simulink model "aa"  (R2021b)
settings: Solver=FixedStepAuto  StartTime=0.0  StopTime=inf  FixedStep=0.00025  RelTol=1e-3  EnableMultiTasking=on
libraries: arduinolib x11, simulink x7, hdlsllib x6
settings Model: ExtModeTrigDuration=2  Creator=user1  LastModifiedBy=ztaha
settings OptimizationCC: EnhancedBackFolding=on  PassReuseOutputArgsThreshold=0  MaxStackSize=64  OptimizeBlockOrder=speed  DifferentSizesBufferReuse=on  OptimizationCustomize=off
settings DebuggingCC: ParameterTunabilityLossMsg=error  UnconnectedInputMsg=none  UnconnectedOutputMsg=none  UnconnectedLineMsg=none
settings HardwareCC: ProdBitPerInt=16  ProdBitPerPointer=16  ProdBitPerSizeT=16  ProdBitPerPtrDiffT=16  ProdLargestAtomicFloat=None  ProdWordSize=8  ProdHWDeviceType=Atmel->AVR  UseEmbeddedCoderFeatures=off  UseSimulinkCoderFeatures=off
settings SFSimCC: MATLABDynamicMemAlloc=off
settings RTWCC: Description=Embedded Coder  SystemTargetFile=ert.tlc  HardwareBoard=Arduino Mega 2560  TemplateMakefile=ert_default_tmf  Toolchain=Arduino AVR  BuildConfiguration=Faster Runs  DLArmComputeVersion=20.02.1
settings CodeAppCC: ForceParamTrailComments=on  OperatorAnnotations=on  MangleLength=10
settings ERTTargetCC: ERTCustomFileBanners=off  SupportContinuousTime=on  SupportNonInlinedSFcns=on  RemoveResetFunc=off  SupportVariableSizeSignals=on  ModelStepFunctionPrototypeControlCompliant=off  ExtModeTransport=3  ExtModeStaticAlloc=on  ExtModeStaticAllocSize=2048  ExtModeMexFile=ext_xcp  ExtModeIntrfLevel=Level2 - Open

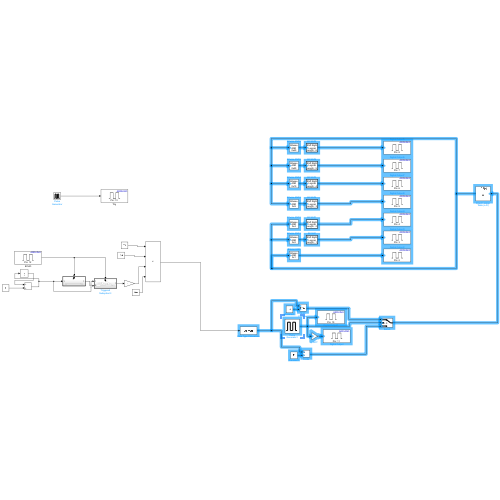
[thumbnail: Simulink's stored preview of the top-level diagram]
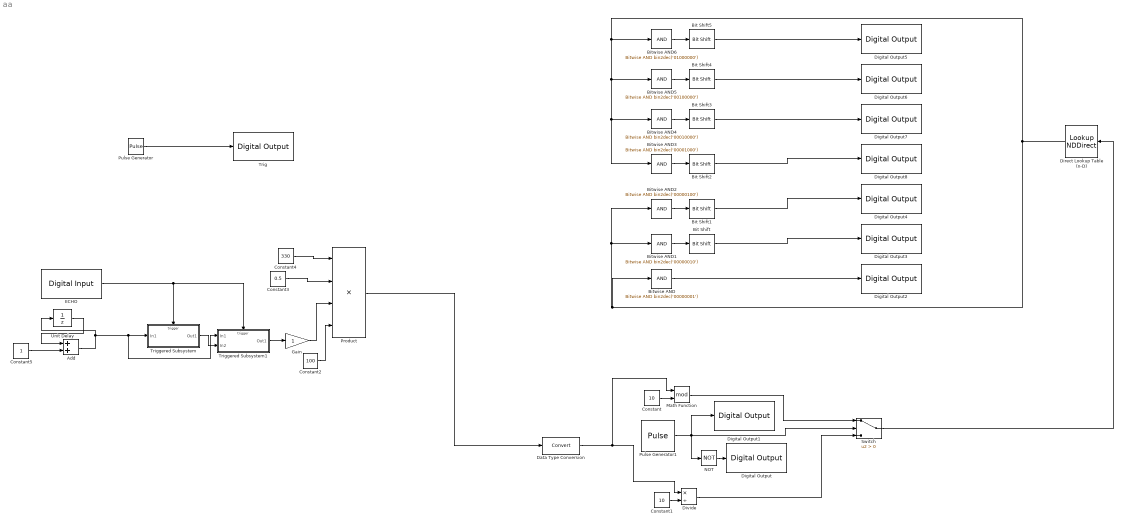
== system aa ==
  Add : Sum
  Bit Shift : hdlsllib/Logic and Bit Operations/Bit Shift  mode=Shift Right Logical  N=1
  Bit Shift1 : hdlsllib/Logic and Bit Operations/Bit Shift  mode=Shift Right Logical  N=2
  Bit Shift2 : hdlsllib/Logic and Bit Operations/Bit Shift  mode=Shift Right Logical  N=3
  Bit Shift3 : hdlsllib/Logic and Bit Operations/Bit Shift  mode=Shift Right Logical  N=4
  Bit Shift4 : hdlsllib/Logic and Bit Operations/Bit Shift  mode=Shift Right Logical  N=5
  Bit Shift5 : hdlsllib/Logic and Bit Operations/Bit Shift  mode=Shift Right Logical  N=6
  Bitwise AND : simulink/Logic and Bit Operations/Bitwise Operator  logicop=AND  UseBitMask=on  BitMask=bin2dec('00000001')  BitMaskRealWorld=Stored Integer
  Bitwise AND1 : simulink/Logic and Bit Operations/Bitwise Operator  logicop=AND  UseBitMask=on  BitMask=bin2dec('00000010')  BitMaskRealWorld=Stored Integer
  Bitwise AND2 : simulink/Logic and Bit Operations/Bitwise Operator  logicop=AND  UseBitMask=on  BitMask=bin2dec('00000100')  BitMaskRealWorld=Stored Integer
  Bitwise AND3 : simulink/Logic and Bit Operations/Bitwise Operator  logicop=AND  UseBitMask=on  BitMask=bin2dec('00001000')  BitMaskRealWorld=Stored Integer
  Bitwise AND4 : simulink/Logic and Bit Operations/Bitwise Operator  logicop=AND  UseBitMask=on  BitMask=bin2dec('00010000')  BitMaskRealWorld=Stored Integer
  Bitwise AND5 : simulink/Logic and Bit Operations/Bitwise Operator  logicop=AND  UseBitMask=on  BitMask=bin2dec('00100000')  BitMaskRealWorld=Stored Integer
  Bitwise AND6 : simulink/Logic and Bit Operations/Bitwise Operator  logicop=AND  UseBitMask=on  BitMask=bin2dec('01000000')  BitMaskRealWorld=Stored Integer
  Constant : Constant  Value=10
  Constant1 : Constant  Value=10
  Constant2 : Constant  Value=100
  Constant3 : Constant  Value=0.5
  Constant4 : Constant  Value=330
  Constant5 : Constant
  Data Type Conversion : DataTypeConversion
  Digital Output : arduinolib/Digital Output  pinNumber=11  Direction=output  blockPlatform=arduino
  Digital Output1 : arduinolib/Digital Output  pinNumber=10  Direction=output  blockPlatform=arduino
  Digital Output2 : arduinolib/Digital Output  pinNumber=2  Direction=output  blockPlatform=arduino
  Digital Output3 : arduinolib/Digital Output  pinNumber=3  Direction=output  blockPlatform=arduino
  Digital Output4 : arduinolib/Digital Output  pinNumber=4  Direction=output  blockPlatform=arduino
  Digital Output5 : arduinolib/Digital Output  pinNumber=8  Direction=output  blockPlatform=arduino
  Digital Output6 : arduinolib/Digital Output  pinNumber=7  Direction=output  blockPlatform=arduino
  Digital Output7 : arduinolib/Digital Output  pinNumber=6  Direction=output  blockPlatform=arduino
  Digital Output8 : arduinolib/Digital Output  pinNumber=5  Direction=output  blockPlatform=arduino
  Direct Lookup Table (n-D) : LookupNDDirect  NumberOfTableDimensions=1  Table=[0xc0; 0xf9; 0xa4; 0xb0; 0x99; 0x92; 0x82; 0xf8; 0x80; 0x90]  TableDataTypeStr=uint8
  Divide : Product  Inputs=*/
  ECHO : arduinolib/Digital Input  pinNumber=12  mode=Default  Direction=input  SampleTime=-1  blockPlatform=arduino
  Gain : Gain
  Math Function : Math  Operator=mod  SaturateOnIntegerOverflow=on
  NOT : Logic  Operator=NOT  IconShape=distinctive  AllPortsSameDT=off  OutDataTypeStr=boolean
  Product : Product  Inputs=4
  Pulse Generator : DiscretePulseGenerator  PulseType=Time based  Period=0.01  PulseWidth=10
  Pulse Generator1 : DiscretePulseGenerator  PulseType=Time based  Period=0.002  PulseWidth=50
  Switch : Switch  Criteria=u2 > Threshold
  Trig : arduinolib/Digital Output  pinNumber=13  Direction=output  blockPlatform=arduino
  Triggered Subsystem : Subsystem  TreatAsAtomicUnit=on
  Triggered Subsystem1 : Subsystem  TreatAsAtomicUnit=on
  Unit Delay : UnitDelay  SampleTime=-1  HasFrameUpgradeWarning=on
  wires:
  Pulse Generator/1 -> Trig/1
  Switch/1 -> Direct Lookup Table (n-D)/1
  Math Function/1 -> Switch/1
  Data Type Conversion/1 -> Divide/1, Math Function/1
  Bitwise AND/1 -> Digital Output2/1
  Bitwise AND4/1 -> Bit Shift3/1
  Bitwise AND6/1 -> Bit Shift5/1
  Constant1/1 -> Divide/2
  Bit Shift2/1 -> Digital Output8/1
  Bitwise AND3/1 -> Bit Shift2/1
  Bit Shift4/1 -> Digital Output6/1
  Bit Shift1/1 -> Digital Output4/1
  Direct Lookup Table (n-D)/1 -> Bitwise AND2/1, Bitwise AND1/1, Bitwise AND/1, Bitwise AND4/1, Bitwise AND3/1, Bitwise AND5/1, Bitwise AND6/1
  Bitwise AND2/1 -> Bit Shift1/1
  Bit Shift3/1 -> Digital Output7/1
  Bit Shift5/1 -> Digital Output5/1
  Bit Shift/1 -> Digital Output3/1
  Constant/1 -> Math Function/2
  Bitwise AND1/1 -> Bit Shift/1
  Divide/1 -> Switch/3
  Bitwise AND5/1 -> Bit Shift4/1
  Pulse Generator1/1 -> Switch/2, Digital Output1/1, NOT/1
  NOT/1 -> Digital Output/1
  Constant4/1 -> Product/1
  Constant3/1 -> Product/2
  ECHO/1 -> Triggered Subsystem1/Trigger, Triggered Subsystem/Trigger
  Triggered Subsystem/1(Out1) -> Triggered Subsystem1/2(In2)
  Unit Delay/1 -> Add/1
  Add/1 -> Triggered Subsystem1/1(In1), Triggered Subsystem/1(In1), Unit Delay/1
  Constant5/1 -> Add/2
  Triggered Subsystem1/1(Out1) -> Gain/1
  Product/1 -> Data Type Conversion/1
  Constant2/1 -> Product/4
  Gain/1 -> Product/3

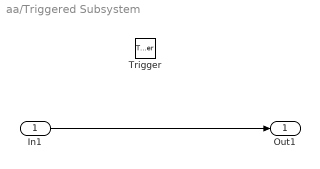
== system aa/Triggered Subsystem ==
  In1 : Inport
  Trigger : TriggerPort  VariantControl=(inherit)
  Out1 : Outport
  wires:
  In1/1 -> Out1/1

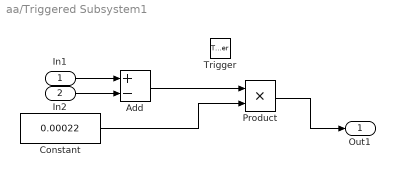
== system aa/Triggered Subsystem1 ==
  In1 : Inport
  In2 : Inport  Port=2
  Trigger : TriggerPort  TriggerType=falling  VariantControl=(inherit)
  Add : Sum  Inputs=+-
  Constant : Constant  Value=0.00022  VectorParams1D=off  SampleTime=-1
  Product : Product
  Out1 : Outport
  wires:
  In1/1 -> Add/1
  In2/1 -> Add/2
  Constant/1 -> Product/2
  Product/1 -> Out1/1
  Add/1 -> Product/1
